simulink model "Att_project_simulink"  (R2022b)
settings: Solver=ode8  StartTime=0.0  StopTime=5000  FixedStep=0.5  RelTol=1e-9  AbsTol=1e-9
values from neighbouring files (symbols this model uses):
  A_R = A_R_BL * ALN_R    [Attitude_proj.m]
  A_T = A_R_BL    [Attitude_proj.m]
  accuracy_earth = deg2rad(10/60)    [Attitude_proj.m]
  accuracy_mag = deg2rad(300/60)    [Attitude_proj.m]
  Cd = 2.3    [Attitude_proj.m]
  I = [Ix 0 0; 0 Iy 0 ; 0 0 Iz]    [Attitude_proj.m]
  Ix = 0.07    [Attitude_proj.m]
  Iy = 0.0504    [Attitude_proj.m]
  Iz = 0.0109    [Attitude_proj.m]
  kd_detum = 2 .* kp_detum    [Attitude_proj.m]
  kd_slew = 2 * kp_slew    [Attitude_proj.m]
  kd_track = kd_detum    [Attitude_proj.m]
  kp_detum = [0.00008 0.0005 0.0005]    [Attitude_proj.m]
  kp_slew = [0.0005 0.0004 0.0004]    [Attitude_proj.m]
  kp_track = kp_detum    [Attitude_proj.m]
  Kx = (Iy-Iz)/Ix    (= 0.564285714286)    [Attitude_proj.m]
  Ky = (Iz-Ix)/Iy    (= -1.17261904762)    [Attitude_proj.m]
  Kz = (Ix-Iy)/Iz    (= 1.79816513761)    [Attitude_proj.m]
  m_para = [0.03;0.04;0.05]    [Attitude_proj.m]
  ortog = (1/3 * deg2rad(1)^2)    [Attitude_proj.m]
  P = Fe/c    (= 4.52980041279e-06)    [Attitude_proj.m]
  q_r = [q1r q2r q3r q4r]    [Attitude_proj.m]
  rho_d_main = 0.1    [Attitude_proj.m]
  rho_d_panel = 0.1    [Attitude_proj.m]
  rho_s_main = 0.5    [Attitude_proj.m]
  rho_s_panel = 0.1    [Attitude_proj.m]
  Rs = 147098074    [Attitude_proj.m]
  w0x = 0.0001    [Attitude_proj.m]
  w0y = orbit.n + 0.005    [Attitude_proj.m]
  w0z = 0.0002    [Attitude_proj.m]
  w_track = [0; orbit.n ; 0]    [Attitude_proj.m]
  zero_w = [ 0; 0; 0]    [Attitude_proj.m]
undefined symbols (not defined in the file or in its folder): body, DiscIntNeverNeededParam, g, h, K, k2, magnitude, orbit, phi0, psi0, theta0, thrus
libraries: vrlib x60, matrix_library x7, simulink x4, sharedutil x4, simulink_extras x2, cstblocks x1, aerolibconvert2 x1, sharedtransform x1
(part 1 of 2)
settings Model: SimulationMode=accelerator  Creator=ASUS  LastModifiedBy=utente
settings SolverCC: ZeroCrossAlgorithm=Adaptive
settings DebuggingCC: AlgebraicLoopMsg=none  MaskedZcDiagnostic=none  IgnoredZcDiagnostic=none  ArithmeticOperatorsInVariantConditions=warning
settings ModelReferenceCC: EnableRefExpFcnMdlSchedulingChecks=on
settings SFSimCC: CustomCodeUndefinedFunction=UseInterfaceOnly
settings RTWCC: DLArmComputeVersion=19.05

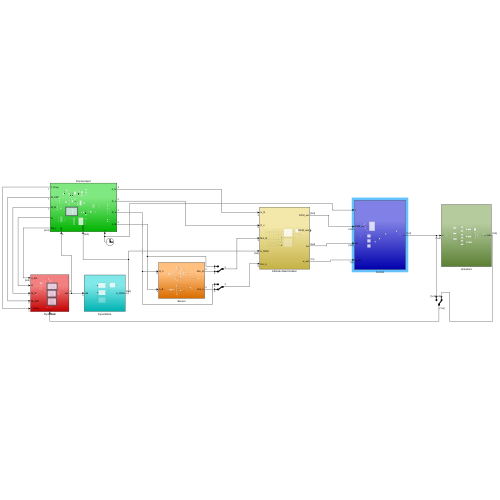
[thumbnail: Simulink's stored preview of the top-level diagram]
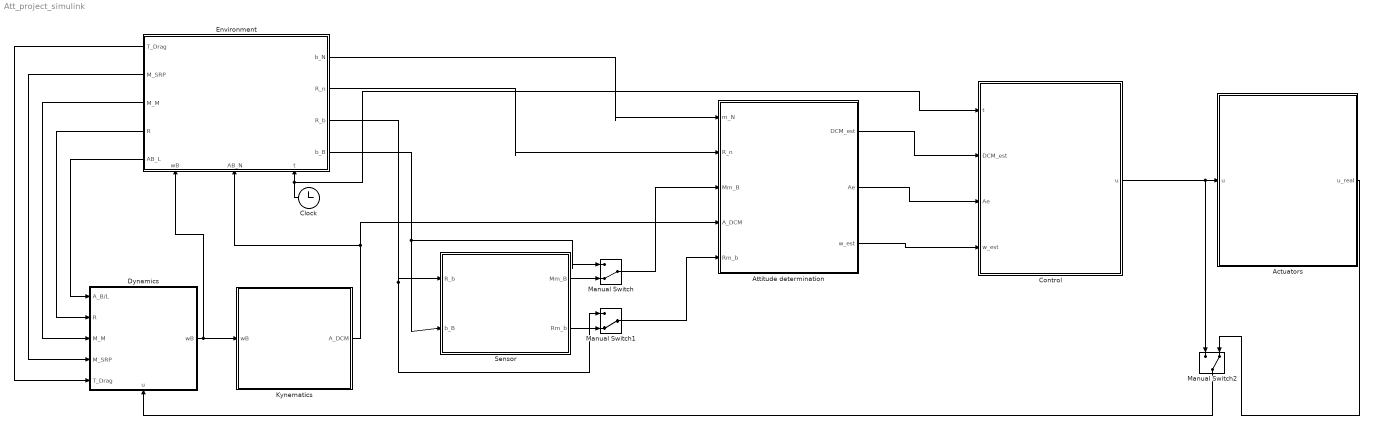
== system Att_project_simulink ==
  Actuators : Subsystem
  Attitude determination : Subsystem
  Clock : Clock
  Control : Subsystem
  Dynamics : Subsystem
      settings: PortSchema="{\"entries\":[{\"content\":{\"sides\":[{\"content\":{\"connectorIds\":[\"In1\",\"In2\",\"In3\",\"In4\",\"In5\"]},\"type\":\"ConnectorPlacement.EquallySpacedRectSide\",\"uuid\":\"e2546f43-0f76-43d8-9016-47189d28d8c0\"},{\"content\":{\"connectorIds\":[\"Out1\"],\"side\":\"RIGHT\"},\"type\":\"ConnectorPlacement.EquallySpacedRectSide\",\"uuid\":\"72ec595a-943a-4b6a-9d51-6626181bb7e6\"},{\"content\":{\"connectorIds\":[],\"side\":\"TOP\"},\"type\":\"ConnectorPlacement.EquallySpacedRectSide\",\"uuid\":\"5bae7898-d8cb-4ebe-a0da-616b512951ce\"},{\"content\":{\"connectorIds\":[\"In6\"],\"side\":\"BOTTOM\"},\"type\":\"ConnectorPlacement.EquallySpacedRectSide\",\"uuid\":\"04644b50-7571-45c4-9210-649b5fcee47a\"}]},\"type\":\"ConnectorPlacement.EquallySpacedConnector\",\"uuid\":\"4d81f698-3eae-4e23-8a75-7ab54dd2047e\"}],\"packageUris\":[\"http://schema.mathworks.com/mf0/Connector/R2020b\"],\"version\":\"1.0\"}"
  Environment : Subsystem
      settings: PortSchema="{\"entries\":[{\"content\":{\"sides\":[{\"content\":{\"connectorIds\":[\"In1\",\"In2\",\"In3\"]},\"type\":\"ConnectorPlacement.EquallySpacedRectSide\",\"uuid\":\"e1717e5b-cb7c-4233-b289-9a3e14a88712\"},{\"content\":{\"connectorIds\":[],\"side\":\"RIGHT\"},\"type\":\"ConnectorPlacement.EquallySpacedRectSide\",\"uuid\":\"74d5df0c-20a5-474c-8972-acb600e0318c\"},{\"content\":{\"connectorIds\":[\"Out5\",\"Out6\",\"Out7\",\"Out8\",\"Out9\"],\"side\":\"TOP\"},\"type\":\"ConnectorPlacement.EquallySpacedRectSide\",\"uuid\":\"8caa1d13-4dab-4013-a60f-fe12337e8062\"},{\"content\":{\"connectorIds\":[\"Out1\",\"Out2\",\"Out3\",\"Out4\"],\"side\":\"BOTTOM\"},\"type\":\"ConnectorPlacement.EquallySpacedRectSide\",\"uuid\":\"a6d0af15-bded-4708-9665-a508da3512a2\"}]},\"type\":\"ConnectorPlacement.EquallySpacedConnector\",\"uuid\":\"6bd2fac6-7248-4b84-8ef8-6b1152c12a45\"}],\"packageUris\":[\"http://schema.mathworks.com/mf0/Connector/R2020b\"],\"version\":\"1.0\"}"
  Kynematics : Subsystem
  Manual Switch : ManualSwitch  CurrentSetting=0
  Manual Switch1 : ManualSwitch  CurrentSetting=0
  Manual Switch2 : ManualSwitch  CurrentSetting=0
  Sensor : Subsystem
  wires:
  Environment/5(AB_L) -> Dynamics/1(A_B/L)
  Environment/6(R) -> Dynamics/2(R)
  Dynamics/1(wB) -> Environment/1(wB), Kynematics/1(wB)
  Environment/7(M_M) -> Dynamics/3(M_M)
  Environment/8(M_SRP) -> Dynamics/4(M_SRP)
  Environment/9(T_Drag) -> Dynamics/5(T_Drag)
  Kynematics/1(A_DCM) -> Environment/2(AB_N), Attitude determination/4(A_DCM)
  Environment/1(b_B) -> Sensor/2(b_B), Manual Switch/1
  Environment/2(R_b) -> Manual Switch1/1, Sensor/1(R_b)
  Sensor/1(Mm_B) -> Manual Switch/2
  Environment/4(b_N) -> Attitude determination/1(m_N)
  Environment/3(R_n) -> Attitude determination/2(R_n)
  Manual Switch/1 -> Attitude determination/3(Mm_B)
  Sensor/2(Rm_b) -> Manual Switch1/2
  Manual Switch1/1 -> Attitude determination/5(Rm_b)
  Clock/1 -> Control/1(t), Environment/3(t)
  Attitude determination/2(Ae) -> Control/3(Ae)
  Control/1(u) -> Manual Switch2/1, Actuators/1(u)
  Attitude determination/1(DCM_est) -> Control/2(DCM_est)
  Attitude determination/3(w_est) -> Control/4(w_est)
  Actuators/1(u_real) -> Manual Switch2/2
  Manual Switch2/1 -> Dynamics/6(u)

== system Att_project_simulink/Actuators ==
  u : Inport
  Demux : Demux  Outputs=3
  If : If
  If Action Subsystem : Subsystem  TreatAsAtomicUnit=on
  If Action Subsystem1 : Subsystem  TreatAsAtomicUnit=on
  If Action Subsystem2 : Subsystem  TreatAsAtomicUnit=on
  If Action Subsystem3 : Subsystem  TreatAsAtomicUnit=on
  If Action Subsystem4 : Subsystem  TreatAsAtomicUnit=on
  If Action Subsystem5 : Subsystem  TreatAsAtomicUnit=on
  If1 : If
  If2 : If
  Merge : Merge
  Merge1 : Merge
  Merge2 : Merge
  Mux : Mux  Inputs=3
  Reshape : Reshape  OutputDimensionality=Customize  OutputDimensions=[1,3]
  Scope : Scope  NumInputPorts=3
  Scope1 : Scope
  To Workspace : ToWorkspace  VariableName=T_c  SaveFormat=Timeseries  SampleTime=-1
  u_real : Outport
  wires:
  u/1 -> Demux/1
  Demux/1 -> If Action Subsystem/1(Mx), If Action Subsystem1/1(-Mx), If/1
  Demux/2 -> If Action Subsystem3/1(-My), If Action Subsystem2/1(My), If1/1
  Demux/3 -> If Action Subsystem5/1(-Mz), If Action Subsystem4/1(Mz), If2/1
  If/1 -> If Action Subsystem/Action
  If/2 -> If Action Subsystem1/Action
  If1/1 -> If Action Subsystem2/Action
  If1/2 -> If Action Subsystem3/Action
  If2/1 -> If Action Subsystem4/Action
  If2/2 -> If Action Subsystem5/Action
  If Action Subsystem4/1(Out1) -> Merge/1  "Z+"
  If Action Subsystem5/1(Out1) -> Merge/2  "Z-"
  If Action Subsystem2/1(Out1) -> Merge1/1  "Y+"
  If Action Subsystem3/1(Out1) -> Merge1/2  "Y-"
  If Action Subsystem/1(Out1) -> Merge2/1  "X+"
  If Action Subsystem1/1(Out1) -> Merge2/2  "X-"
  Mux/1 -> Reshape/1
  Reshape/1 -> Scope1/1, To Workspace/1, u_real/1
  Merge2/1 -> Scope/1, Mux/1
  Merge1/1 -> Scope/2, Mux/2
  Merge/1 -> Scope/3, Mux/3

== system Att_project_simulink/Attitude determination ==
  m_N : Inport
  R_n : Inport  Port=2
  Mm_B : Inport  Port=3
  A_DCM : Inport  Port=4
  Rm_b : Inport  Port=5
  Triad Method : Subsystem
  w_esti : Subsystem
  DCM_est : Outport
  Ae : Outport  Port=2
  w_est : Outport  Port=3
  wires:
  A_DCM/1 -> Triad Method/5(A_DCM)
  Rm_b/1 -> Triad Method/1(Rm_b)
  m_N/1 -> Triad Method/4(m_N)
  Mm_B/1 -> Triad Method/3(Mm_B)
  R_n/1 -> Triad Method/2(R_n)
  Triad Method/1(DCM_est) -> DCM_est/1, w_esti/1(DCM_est)
  Triad Method/2(Ae) -> Ae/1
  w_esti/1(Output) -> w_est/1

== system Att_project_simulink/Control ==
  t : Inport
  DCM_est : Inport  Port=2
  Ae : Inport  Port=3
  w_est : Inport  Port=4
  De-tumbling : Subsystem  Commented=on
  Manual Switch : ManualSwitch  CurrentSetting=0
  Manual Switch1 : ManualSwitch  CurrentSetting=0
  Manual Switch2 : ManualSwitch
  Scope : Scope
  Tracking : Subsystem
  ble : Subsystem  Commented=on
  slew : Subsystem  Commented=on
  w_est1 : InportShadow  Port=4
  u : Outport
  wires:
  Ae/1 -> slew/1(Ae), Tracking/1(Ae), ble/1(Ae)
  [wB] -> ?
  t/1 -> ble/2(t)
  w_est/1 -> ble/3(w_est)
  DCM_est/1 -> ble/4(DCM_est)
  ble/1(u) -> Manual Switch/1
  Manual Switch/1 -> Scope/1, u/1
  w_est1/1 -> De-tumbling/1(In1)
  De-tumbling/1(Out1) -> Manual Switch1/1
  Tracking/1(u) -> Manual Switch2/1
  Manual Switch1/1 -> Manual Switch/2
  slew/1(u) -> Manual Switch2/2
  Manual Switch2/1 -> Manual Switch1/2

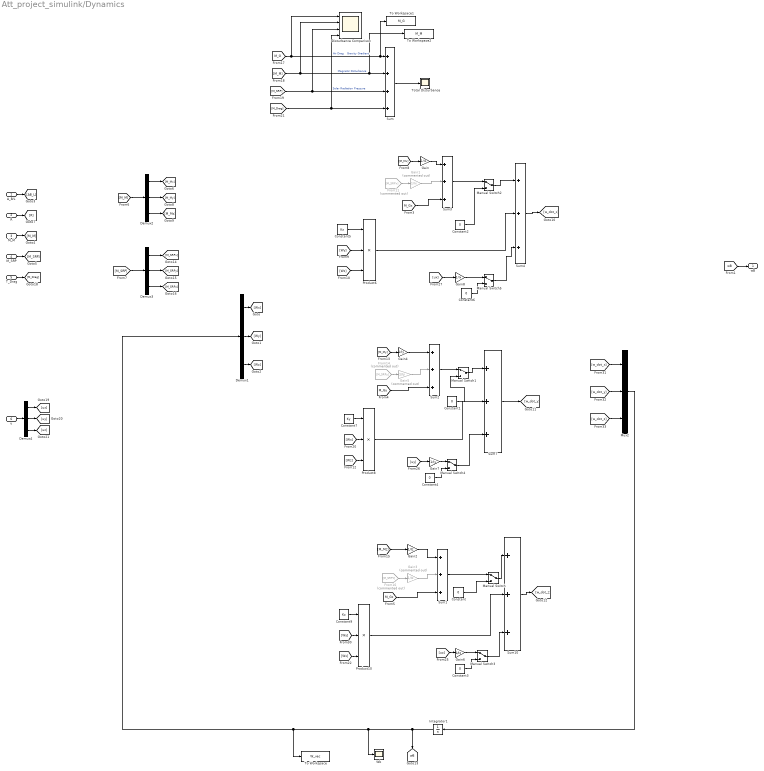
== system Att_project_simulink/Dynamics ==
  A_B/L : Inport
  R : Inport  Port=2
  M_M : Inport  Port=3
  M_SRP : Inport  Port=4
  T_Drag : Inport  Port=5
  u : Inport  Port=6
  Constant{,1..4,6} (6 alike) : Constant  Value=0
  Constant5 : Constant  Value=Kx
  Constant7 : Constant  Value=Ky
  Constant9 : Constant  Value=Kz
  Demux{1..4} (4 alike) : Demux  Outputs=3
  Disturbance Comparison : Scope  NumInputPorts=4
  From11 : From  Commented=on  GotoTag=M_SRPx
  From14 : From  Commented=on  GotoTag=M_SRPy
  From16 : From  Commented=on  GotoTag=M_SRPz
  Gain : Gain  Gain=1/Ix
  Gain1 : Gain  Commented=on  Gain=1/Ix
  Gain2 : Gain  Gain=1/Iz
  Gain3 : Gain  Commented=on  Gain=1/Iz
  Gain4 : Gain  Gain=1/Iy
  Gain5 : Gain  Commented=on  Gain=1/Iy
  Gain6 : Gain  Gain=1/Iz
  Gain7 : Gain  Gain=1/Iy
  Gain8 : Gain  Gain=1/Ix
  Integrator1 : Integrator  InitialCondition=[w0x; w0y; w0z]'
  Manual Switch{,1..5} (6 alike) : ManualSwitch
  Mux2 : Mux  Inputs=3
  Product10 : Product  Inputs=3
  Product6 : Product  Inputs=3
  Product8 : Product  Inputs=3
  Sum : Sum  Inputs=++++
  Sum{1..4,7,10} (6 alike) : Sum  Inputs=+++
  To Workspace : ToWorkspace  VariableName=W_vec  SaveFormat=Timeseries  SampleTime=-1
  To Workspace1 : ToWorkspace  VariableName=M_G  SaveFormat=Timeseries  SampleTime=-1
  To Workspace2 : ToWorkspace  VariableName=M_M  SaveFormat=Timeseries  SampleTime=-1
  Total Disturbance : Scope
  Wb : Scope
  wB : Outport
  tag scope: wB=global
  wires:
  Demux1/3 -> [Wz]
  Demux1/2 -> [Wy]
  Demux1/1 -> [Wx]
  A_B/L/1 -> [AB_L]
  [Wy] -> Product6/2
  [Wz] -> Product6/3
  Product6/1 -> Sum4/2
  Sum4/1 -> [w_dot_x]
  Product8/1 -> Sum7/2
  [Wx] -> Product8/2
  Sum7/1 -> [w_dot_y]
  [Wz] -> Product8/3
  Product10/1 -> Sum10/2
  [Wy] -> Product10/2
  Constant9/1 -> Product10/1
  Sum10/1 -> [w_dot_z]
  [Wx] -> Product10/3
  [w_dot_z] -> Mux2/3
  [w_dot_y] -> Mux2/2
  [w_dot_x] -> Mux2/1
  Integrator1/1 -> Wb/1, To Workspace/1, Demux1/1, [wB]
  Constant5/1 -> Product6/1
  Constant7/1 -> Product8/1
  [wB] -> wB/1
  R/1 -> [R]
  M_M/1 -> [M_M]
  M_SRP/1 -> [M_SRP]
  Demux2/1 -> [M_Mx]
  Demux2/2 -> [M_My]
  Demux2/3 -> [M_Mz]
  [M_M] -> Demux2/1
  Demux3/2 -> [M_SRPy]
  Demux3/1 -> [M_SRPx]
  [M_SRP] -> Demux3/1
  Demux3/3 -> [M_SRPz]
  [M_Mx] -> Gain/1
  From11/1 -> Gain1/1
  [M_My] -> Gain4/1
  From14/1 -> Gain5/1
  From16/1 -> Gain3/1
  [M_Mz] -> Gain2/1
  [M_SRP] -> Sum/3, Disturbance Comparison/3  "Solar Radiation Pressure"
  [M_M] -> To Workspace2/1, Sum/2, Disturbance Comparison/2  "Magnetic Disturbance"
  [M_G] -> Disturbance Comparison/1, To Workspace1/1, Sum/1  "Gravity Gradient"
  Sum/1 -> Total Disturbance/1
  T_Drag/1 -> [M_Drag]
  [M_Drag] -> Sum/4, Disturbance Comparison/4  "Air Drag"
  Gain2/1 -> Sum1/1
  Gain3/1 -> Sum1/2
  [M_Gz] -> Sum1/3
  Sum1/1 -> Manual Switch/1
  Constant/1 -> Manual Switch/2
  Gain4/1 -> Sum2/1
  Gain5/1 -> Sum2/2
  [M_Gy] -> Sum2/3
  Sum2/1 -> Manual Switch1/1
  Manual Switch1/1 -> Sum7/1
  Constant1/1 -> Manual Switch1/2
  Manual Switch/1 -> Sum10/1
  Gain1/1 -> Sum3/2
  Gain/1 -> Sum3/1
  [M_Gx] -> Sum3/3
  Sum3/1 -> Manual Switch2/1
  Manual Switch2/1 -> Sum4/1
  Constant2/1 -> Manual Switch2/2
  Manual Switch3/1 -> Sum10/3
  Constant3/1 -> Manual Switch3/2
  u/1 -> Demux4/1
  Demux4/1 -> [ux]
  Demux4/2 -> [uy]
  Demux4/3 -> [uz]
  [uz] -> Gain6/1
  Constant4/1 -> Manual Switch4/2
  Manual Switch4/1 -> Sum7/3
  [uy] -> Gain7/1
  Constant6/1 -> Manual Switch5/2
  Manual Switch5/1 -> Sum4/3
  [ux] -> Gain8/1
  Gain6/1 -> Manual Switch3/1
  Gain7/1 -> Manual Switch4/1
  Gain8/1 -> Manual Switch5/1
  Mux2/1 -> Integrator1/1

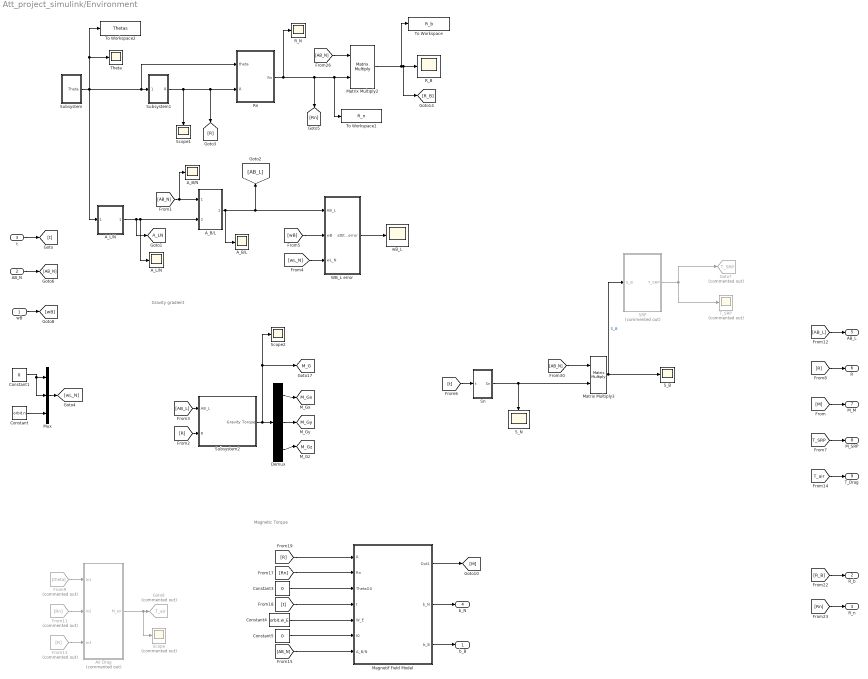
== system Att_project_simulink/Environment ==
  note: Gravity gradient
  note: Magnetic Torque
  wB : Inport
  AB_N : Inport  Port=2
  t : Inport  Port=3
  A_B/L : Scope
  "A_B/L " : Subsystem
  A_B/N : Scope
  A_L/N : Scope
  "A_L/N " : Subsystem
  "Air Drag " : Subsystem  Commented=on
  Constant : Constant  Value=orbit.n
  Constant1 : Constant  Value=0
  Constant3 : Constant  Value=0
  Constant4 : Constant  Value=orbit.w_E
  Constant5 : Constant  Value=0
  Demux : Demux  Outputs=3
  From11 : From  Commented=on  GotoTag=Rn
  From13 : From  Commented=on  GotoTag=R
  From9 : From  Commented=on  GotoTag=theta
  Goto7 : Goto  Commented=on  GotoTag=T_SRP  TagVisibility=global
  Goto9 : Goto  Commented=on  GotoTag=T_air  TagVisibility=global
  Magnetif Field Model : Subsystem
  Matrix Multiply2 : Product  Multiplication=Matrix(*)
  Matrix Multiply3 : Product  Multiplication=Matrix(*)
  Mux : Mux  Inputs=3
  R_B : Scope
  R_N : Scope
  Rn : Subsystem
  SRP : Subsystem  Commented=on
  S_B : Scope
  S_N : Scope
  Scope : Scope  Commented=on
  Scope1 : Scope
  Scope2 : Scope
  Sn : Subsystem
  Subsystem : Subsystem
  Subsystem1 : Subsystem
  Subsystem2 : Subsystem
  T_SRP : Scope  Commented=on
  Theta : Scope
  To Workspace : ToWorkspace  VariableName=R_b  SaveFormat=Timeseries  SampleTime=-1
  To Workspace1 : ToWorkspace  VariableName=R_n  SaveFormat=Timeseries  SampleTime=-1
  To Workspace2 : ToWorkspace  VariableName=Thetas  SaveFormat=Timeseries  SampleTime=-1
  WB_L error : Subsystem
  wB_L : Scope
  b_B : Outport
  R_b : Outport  Port=2
  R_n : Outport  Port=3
  b_N : Outport  Port=4
  AB_L : Outport  Port=5
  R : Outport  Port=6
  M_M : Outport  Port=7
  M_SRP : Outport  Port=8
  T_Drag : Outport  Port=9
  tag scope: A_LN=global, M_G=global, M_Gx=global, M_Gy=global, M_Gz=global
  wires:
  t/1 -> [t]
  Constant/1 -> Mux/3
  Mux/1 -> [wL_N]
  AB_N/1 -> [AB_N]
  [AB_L] -> AB_L/1
  Matrix Multiply2/1 -> To Workspace/1, [R_B], R_B/1
  Subsystem/1(Theta) -> Rn/1(theta), Subsystem1/1(Theta), To Workspace2/1, Theta/1, "A_L/N "/1(theta)
  [AB_N] -> A_B/N/1, "A_B/L "/1(AB_N)
  "A_L/N "/1(AL_N) -> [A_LN], "A_B/L "/2(AL_N), A_L/N/1
  WB_L error/1(attitude error) -> wB_L/1
  "A_B/L "/1(AB_L) -> A_B/L/1, WB_L error/1(AB_L), [AB_L]
  [wL_N] -> WB_L error/3(wL_N)
  Subsystem1/1(R) -> Scope1/1, Rn/2(R), [R]
  [R] -> R/1
  Rn/1(Rn) -> R_N/1, To Workspace1/1, Matrix Multiply2/2, [Rn]
  [AB_N] -> Matrix Multiply2/1
  Constant1/1 -> Mux/2, Mux/1
  wB/1 -> [wB]
  [wB] -> WB_L error/2(wB)
  [T_SRP] -> M_SRP/1
  [M] -> M_M/1
  From9/1 -> "Air Drag "/1(In1)
  From11/1 -> "Air Drag "/2(In2)
  From13/1 -> "Air Drag "/3(In3)
  "Air Drag "/1(M_air) -> Scope/1, Goto9/1
  [T_air] -> T_Drag/1
  [Rn] -> Magnetif Field Model/2(Rn)
  Constant3/1 -> Magnetif Field Model/3(ThetaG0)
  [t] -> Magnetif Field Model/4(t)
  Constant4/1 -> Magnetif Field Model/5(W_E)
  Constant5/1 -> Magnetif Field Model/6(t0)
  [AB_N] -> Magnetif Field Model/7(A_B/N)
  [R] -> Magnetif Field Model/1(R)
  Magnetif Field Model/1(Out1) -> [M]
  [t] -> Sn/1(t)
  Sn/1(Sn) -> Matrix Multiply3/2, S_N/1
  Matrix Multiply3/1 -> SRP/1(S_B), S_B/1  "S_B"
  SRP/1(T_SRP) -> T_SRP/1, Goto7/1
  [AB_N] -> Matrix Multiply3/1
  Magnetif Field Model/2(b_N) -> b_N/1
  Magnetif Field Model/3(b_B) -> b_B/1
  [R_B] -> R_b/1
  [Rn] -> R_n/1
  [R] -> Subsystem2/2(R)
  Subsystem2/1(Gravity Torque) -> Scope2/1, [M_G], Demux/1
  Demux/2 -> [M_Gy]
  Demux/3 -> [M_Gz]
  [AB_L] -> Subsystem2/1(AB_L)
  Demux/1 -> [M_Gx]

== system Att_project_simulink/Kynematics ==
  wB : Inport
  DCM : Subsystem
  Euler Angles : Subsystem  Commented=on
  From Quat to DCM : Subsystem
  Quaternions : Subsystem
  A_DCM : Outport
  wires:
  Quaternions/1(q(t)) -> From Quat to DCM/1(q(t))
  From Quat to DCM/1(A_DCM) -> A_DCM/1
  wB/1 -> Euler Angles/1(wB), DCM/1(wB), Quaternions/1(wB)
  DCM/1(dcm) -> From Quat to DCM/2(dcm)

== system Att_project_simulink/Sensor ==
  R_b : Inport
  b_B : Inport  Port=2
  Demux : Demux  Outputs=3
  Demux1 : Demux  Outputs=3
  Mux : Mux  Inputs=3
  Mux1 : Mux  Inputs=3
  Normalize Vector : vrlib/Utilities/Normalize Vector  maxzero=0
  Normalize Vector1 : vrlib/Utilities/Normalize Vector  maxzero=0
  Random Number1 : RandomNumber  Variance=(1/3*accuracy_mag).^2  Seed=1  SampleTime=1
  Random Number10 : RandomNumber  Variance=ortog  Seed=2  SampleTime=2
  Random Number11 : RandomNumber  Variance=ortog  Seed=3  SampleTime=2
  Random Number2 : RandomNumber  Variance=(1/3*accuracy_mag).^2  Seed=2  SampleTime=1
  Random Number3 : RandomNumber  Variance=(1/3*accuracy_mag).^2  Seed=3  SampleTime=1
  Random Number4 : RandomNumber  Variance=(1/3*accuracy_earth).^2  Seed=4  SampleTime=2
  Random Number7 : RandomNumber  Variance=(1/3*accuracy_earth).^2  Seed=5  SampleTime=2
  Random Number8 : RandomNumber  Variance=(1/3*accuracy_earth).^2  Seed=6  SampleTime=2
  Random Number9 : RandomNumber  Variance=ortog  Seed=1  SampleTime=2
  Reshape : Reshape  OutputDimensionality=Customize  OutputDimensions=[3,1]
  Reshape1 : Reshape  OutputDimensionality=Customize  OutputDimensions=[3,1]
  Scope3 : Scope  NumInputPorts=2
  Scope4 : Scope  NumInputPorts=2
  Sum1 : Sum  Inputs=+++
  Sum2 : Sum  Inputs=+++
  Sum3 : Sum  Inputs=+++
  Sum4 : Sum  Inputs=++|
  Sum5 : Sum  Inputs=|++
  Sum6 : Sum  Inputs=|++
  Mm_B : Outport
  Rm_b : Outport  Port=2
  wires:
  Random Number1/1 -> Sum1/1
  Demux/3 -> Sum3/1
  Random Number3/1 -> Sum3/2
  Sum1/1 -> Mux/1
  Sum2/1 -> Mux/2
  Sum3/1 -> Mux/3
  Demux1/2 -> Sum5/1
  Random Number7/1 -> Sum5/2
  Demux1/3 -> Sum6/1
  Random Number8/1 -> Sum6/2
  Random Number4/1 -> Sum4/1
  Sum4/1 -> Mux1/1
  Sum6/1 -> Mux1/3
  Demux1/1 -> Sum4/2
  Sum5/1 -> Mux1/2
  Mux1/1 -> Scope3/2, Rm_b/1
  R_b/1 -> Normalize Vector/1
  Normalize Vector/1 -> Reshape1/1
  Normalize Vector1/1 -> Reshape/1
  Mux/1 -> Mm_B/1, Scope4/1
  b_B/1 -> Normalize Vector1/1
  Demux/1 -> Sum1/3
  Random Number9/1 -> Sum1/2
  Random Number2/1 -> Sum2/1
  Random Number10/1 -> Sum2/2
  Demux/2 -> Sum2/3
  Random Number11/1 -> Sum3/3
  Reshape/1 -> Scope4/2, Demux/1
  Reshape1/1 -> Scope3/1, Demux1/1

== system Att_project_simulink/Actuators/If Action Subsystem ==
  Mx : Inport
  Action Port : ActionPort  ActionPortLabel=if(u1 > 0)
  Abs : Abs  SaturateOnIntegerOverflow=off
  Constant : Constant  Value=thrus.ACT_x1(3)
  Divide : Product  Inputs=*/
  Product : Product
  Saturation : Saturate  UpperLimit=thrus.up_sat  LowerLimit=thrus.low_sat
  Out1 : Outport
  wires:
  Mx/1 -> Divide/1
  Constant/1 -> Abs/1
  Divide/1 -> Saturation/1
  Saturation/1 -> Product/2
  Product/1 -> Out1/1
  Abs/1 -> Product/1, Divide/2

== system Att_project_simulink/Actuators/If Action Subsystem1 ==
  -Mx : Inport
  Action Port : ActionPort  ActionPortLabel=else
  Abs : Abs  SaturateOnIntegerOverflow=off
  Constant : Constant  Value=thrus.ACT_x2(3)
  Divide : Product  Inputs=*/
  Gain : Gain  Gain=-1
  Gain1 : Gain  Gain=-1
  Product : Product
  Saturation : Saturate  UpperLimit=thrus.up_sat  LowerLimit=thrus.low_sat
  Scope : Scope  NumInputPorts=2
  Out1 : Outport
  wires:
  Saturation/1 -> Scope/2, Product/2
  Product/1 -> Gain1/1
  Constant/1 -> Abs/1
  Divide/1 -> Scope/1, Saturation/1
  -Mx/1 -> Gain/1
  Abs/1 -> Product/1, Divide/2
  Gain/1 -> Divide/1
  Gain1/1 -> Out1/1

== system Att_project_simulink/Actuators/If Action Subsystem2 ==
  My : Inport
  Action Port : ActionPort  ActionPortLabel=if(u1 > 0)
  Abs : Abs  SaturateOnIntegerOverflow=off
  Constant : Constant  Value=thrus.ACT_y1(3)
  Divide : Product  Inputs=*/
  Product : Product
  Saturation : Saturate  UpperLimit=thrus.up_sat  LowerLimit=thrus.low_sat
  Out1 : Outport
  wires:
  Saturation/1 -> Product/2
  Product/1 -> Out1/1
  Constant/1 -> Abs/1
  Divide/1 -> Saturation/1
  My/1 -> Divide/1
  Abs/1 -> Product/1, Divide/2

== system Att_project_simulink/Actuators/If Action Subsystem3 ==
  -My : Inport
  Action Port : ActionPort  ActionPortLabel=else
  Abs : Abs  SaturateOnIntegerOverflow=off
  Constant : Constant  Value=thrus.ACT_y2(3)
  Divide : Product  Inputs=*/
  Gain : Gain  Gain=-1
  Gain1 : Gain  Gain=-1
  Product : Product
  Saturation : Saturate  UpperLimit=thrus.up_sat  LowerLimit=thrus.low_sat
  Out1 : Outport
  wires:
  Saturation/1 -> Product/2
  Product/1 -> Gain1/1
  Constant/1 -> Abs/1
  Divide/1 -> Saturation/1
  -My/1 -> Gain/1
  Abs/1 -> Product/1, Divide/2
  Gain/1 -> Divide/1
  Gain1/1 -> Out1/1

== system Att_project_simulink/Actuators/If Action Subsystem4 ==
  Mz : Inport
  Action Port : ActionPort  ActionPortLabel=if(u1 > 0)
  Abs : Abs  SaturateOnIntegerOverflow=off
  Constant : Constant  Value=thrus.ACT_z1(2)
  Divide : Product  Inputs=*/
  Product : Product
  Saturation : Saturate  UpperLimit=thrus.up_sat  LowerLimit=thrus.low_sat
  Out1 : Outport
  wires:
  Saturation/1 -> Product/2
  Product/1 -> Out1/1
  Constant/1 -> Abs/1
  Divide/1 -> Saturation/1
  Mz/1 -> Divide/1
  Abs/1 -> Product/1, Divide/2

== system Att_project_simulink/Actuators/If Action Subsystem5 ==
  -Mz : Inport
  Action Port : ActionPort  ActionPortLabel=else
  Abs : Abs  SaturateOnIntegerOverflow=off
  Constant : Constant  Value=thrus.ACT_z2(2)
  Divide : Product  Inputs=*/
  Gain : Gain  Gain=-1
  Gain1 : Gain  Gain=-1
  Product : Product
  Saturation : Saturate  UpperLimit=thrus.up_sat  LowerLimit=thrus.low_sat
  Out1 : Outport
  wires:
  Saturation/1 -> Product/2
  Product/1 -> Gain1/1
  Constant/1 -> Abs/1
  Divide/1 -> Saturation/1
  -Mz/1 -> Gain/1
  Abs/1 -> Product/1, Divide/2
  Gain/1 -> Divide/1
  Gain1/1 -> Out1/1

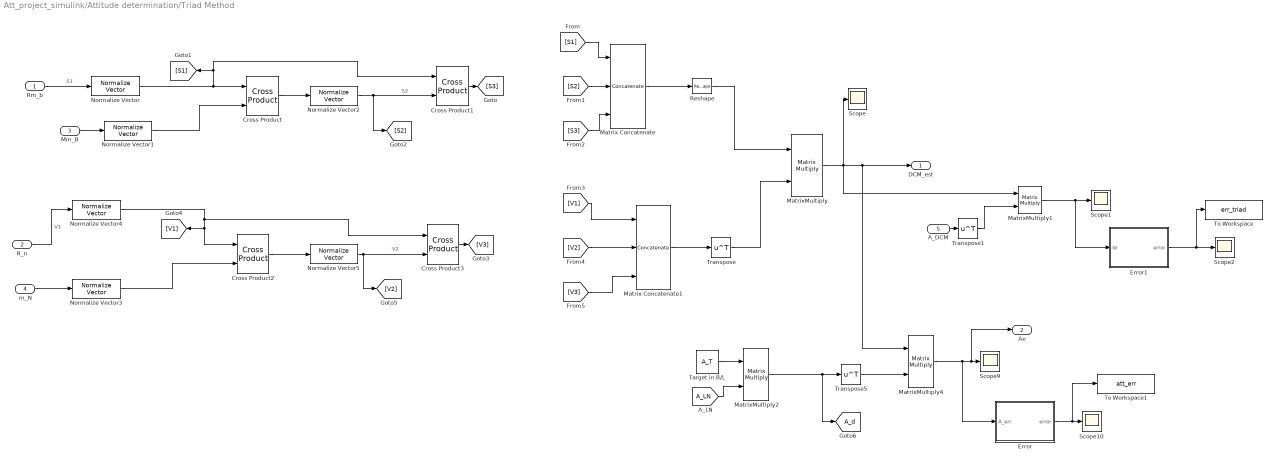
== system Att_project_simulink/Attitude determination/Triad Method ==
  Rm_b : Inport
  R_n : Inport  Port=2
  Mm_B : Inport  Port=3
  m_N : Inport  Port=4
  A_DCM : Inport  Port=5
  Cross Product{,1..3} (4 alike) : matrix_library/Cross Product
  Error : Subsystem
  Error1 : Subsystem
  Matrix Concatenate : Concatenate  NumInputs=3  Mode=Multidimensional array  ConcatenateDimension=2
  Matrix Concatenate1 : Concatenate  NumInputs=3  Mode=Multidimensional array  ConcatenateDimension=2
  MatrixMultiply{,1..2,4} (4 alike) : Product  Multiplication=Matrix(*)
  Normalize Vector{,1..5} (6 alike) : vrlib/Utilities/Normalize Vector  maxzero=0
  Reshape : Reshape  OutputDimensionality=Customize  OutputDimensions=[3,3]
  Scope{,1..2,9..10} (5 alike) : Scope
  Target in B/L : Constant  Value=A_T  VectorParams1D=off
  To Workspace : ToWorkspace  VariableName=err_triad  SaveFormat=Structure  SampleTime=-1
  To Workspace1 : ToWorkspace  VariableName=att_err  SaveFormat=Timeseries  SampleTime=-1
  Transpose : Math  Operator=transpose
  Transpose1 : Math  Operator=transpose
  Transpose5 : Math  Operator=transpose
  DCM_est : Outport
  Ae : Outport  Port=2
  tag scope: A_d=global
  wires:
  Rm_b/1 -> Normalize Vector/1  "S1"
  Cross Product/1 -> Normalize Vector2/1
  Normalize Vector2/1 -> [S2], Cross Product1/2  "S2"
  Cross Product1/1 -> [S3]
  m_N/1 -> Normalize Vector3/1
  Cross Product3/1 -> [V3]
  Cross Product2/1 -> Normalize Vector5/1
  R_n/1 -> Normalize Vector4/1  "V1"
  Normalize Vector5/1 -> [V2], Cross Product3/2  "V2"
  [S1] -> Matrix Concatenate/1
  [S2] -> Matrix Concatenate/2
  [S3] -> Matrix Concatenate/3
  [V1] -> Matrix Concatenate1/1
  [V2] -> Matrix Concatenate1/2
  [V3] -> Matrix Concatenate1/3
  Matrix Concatenate1/1 -> Transpose/1
  Transpose/1 -> MatrixMultiply/2
  MatrixMultiply/1 -> DCM_est/1, MatrixMultiply4/1, MatrixMultiply1/1, Scope/1
  A_DCM/1 -> Transpose1/1
  Transpose1/1 -> MatrixMultiply1/2
  MatrixMultiply1/1 -> Error1/1(Id), Scope1/1
  Normalize Vector/1 -> [S1], Cross Product1/1, Cross Product/1
  Mm_B/1 -> Normalize Vector1/1
  Normalize Vector1/1 -> Cross Product/2
  Normalize Vector4/1 -> Cross Product2/1, [V1], Cross Product3/1
  Normalize Vector3/1 -> Cross Product2/2
  Transpose5/1 -> MatrixMultiply4/2
  MatrixMultiply4/1 -> Error/1(A_err), Ae/1, Scope9/1
  Error/1(error) -> To Workspace1/1, Scope10/1
  Error1/1(error) -> To Workspace/1, Scope2/1
  Target in B/L/1 -> MatrixMultiply2/1
  [A_LN] -> MatrixMultiply2/2
  Matrix Concatenate/1 -> Reshape/1
  Reshape/1 -> MatrixMultiply/1
  MatrixMultiply2/1 -> [A_d], Transpose5/1

== system Att_project_simulink/Attitude determination/w_esti ==
  DCM_est : Inport
  Constant : Constant  Value=0.2
  Discrete Derivative : simulink/Quick Insert/Discrete/Discrete Derivative  gainval=1.0  ICPrevScaledInput=0.0  OutMin=[]  OutMax=[]  OutDataType=fixdt(1, 16)  OutScaling=2^-10  DoSatur=off
  Discrete Varying Lowpass : cstblocks/Linear Parameter Varying/Discrete Varying Lowpass  N=5  w0=0  Ts=1
  Gain : Gain  Gain=-1
  MATLAB Function : MATLAB Function  TreatAsAtomicUnit=on
  Manual Switch1 : ManualSwitch
  MatrixMultiply : Product  Multiplication=Matrix(*)
  Scope : Scope  NumInputPorts=2
  Scope1 : Scope
  Scope2 : Scope
  Sum : Sum  Inputs=|+-
  Transpose : Math  Operator=transpose
  Output : Outport
  wires:
  DCM_est/1 -> Discrete Derivative/1, Transpose/1
  [wB] -> Scope2/1, Scope/2, Sum/2
  Sum/1 -> Scope1/1
  Gain/1 -> MATLAB Function/1(w)
  MatrixMultiply/1 -> Gain/1  "-w"
  Discrete Derivative/1 -> MatrixMultiply/1
  Transpose/1 -> MatrixMultiply/2
  MATLAB Function/1(w_est) -> Manual Switch1/2, Discrete Varying Lowpass/1
  Discrete Varying Lowpass/1 -> Manual Switch1/1
  Manual Switch1/1 -> Sum/1, Output/1, Scope/1
  Constant/1 -> Discrete Varying Lowpass/2

== system Att_project_simulink/Control/De-tumbling ==
  In1 : Inport
  Constant : Constant  Value=zero_w
  Discrete Derivative : simulink/Discrete/Discrete Derivative  gainval=1.0  ICPrevScaledInput=0.0  OutMin=[]  OutMax=[]  OutDataType=fixdt(1, 16)  OutScaling=2^-10  DoSatur=off
  Discrete-Time Integrator : DiscreteIntegrator  SampleTime=-1  ICPrevOutput=DiscIntNeverNeededParam  ICPrevScaledInput=DiscIntNeverNeededParam
  Gain : Gain  Gain=-kp_detum
  Gain1 : Gain  Gain=-kd_detum
  Gain2 : Gain  Gain=-kp_detum
  Reshape : Reshape  OutputDimensionality=Customize  OutputDimensions=[1,3]
  Reshape1 : Reshape  OutputDimensionality=Customize  OutputDimensions=[1,3]
  Sum : Sum  Inputs=+++
  Sum1 : Sum  Inputs=|++
  Out1 : Outport
  wires:
  In1/1 -> Reshape/1
  Discrete Derivative/1 -> Gain1/1
  Sum/1 -> Reshape1/1
  Reshape/1 -> Discrete-Time Integrator/1, Gain/1, Discrete Derivative/1
  Reshape1/1 -> Out1/1
  Gain/1 -> Sum1/1
  Constant/1 -> Sum1/2
  Sum1/1 -> Sum/2
  Gain1/1 -> Sum/3
  Discrete-Time Integrator/1 -> Gain2/1
  Gain2/1 -> Sum/1

== system Att_project_simulink/Control/Tracking ==
  Ae : Inport
  Constant : Constant  Value=w_track
  Discrete Derivative : simulink/Discrete/Discrete Derivative  gainval=1.0  ICPrevScaledInput=0.0  OutMin=[]  OutMax=[]  OutDataType=fixdt(1, 16)  OutScaling=2^-10  DoSatur=off
  Gain : Gain  Gain=-kp_track
  Gain1 : Gain  Gain=-kd_track
  Mux : Mux  Inputs=3
  Scope : Scope
  Selector : Selector  NumberOfDimensions=2  InputPortWidth=3  IndexOptions=Index vector (dialog),Index vector (dialog)  Indices=2,3  OutputSizes=1,1
  Selector1 : Selector  NumberOfDimensions=2  InputPortWidth=3  IndexOptions=Index vector (dialog),Index vector (dialog)  Indices=3,1  OutputSizes=1,1
  Selector2 : Selector  NumberOfDimensions=2  InputPortWidth=3  IndexOptions=Index vector (dialog),Index vector (dialog)  Indices=1,2  OutputSizes=1,1
  Sum : Sum  Inputs=|++
  Sum1 : Sum  Inputs=|+-
  u : Outport
  wires:
  Selector/1 -> Mux/1
  Selector2/1 -> Mux/3
  Gain1/1 -> Sum/1
  Gain/1 -> Sum/2
  Selector1/1 -> Mux/2
  Discrete Derivative/1 -> Sum1/1, Scope/1
  Constant/1 -> Sum1/2
  Sum1/1 -> Gain1/1
  Mux/1 -> Gain/1, Discrete Derivative/1
  Sum/1 -> u/1
  Ae/1 -> Selector/1, Selector2/1, Selector1/1

== system Att_project_simulink/Control/ble ==
  Ae : Inport
  t : Inport  Port=2
  w_est : Inport  Port=3
  DCM_est : Inport  Port=4
  Constant1 : Constant  Value=I
  Demux : Demux  Outputs=9
  Extract Diagonal : matrix_library/Extract Diagonal
      settings: LibrarySourceBlock=|
      | simulink/Matrix
      | Operations/Extract Diagonal
  Gain1 : Gain  Gain=k2
  Gain2 : Gain  Gain=-kd_track
  Gain3 : Gain  Gain=-kp_track
  Gain4 : Gain  Gain=0.5
  MatrixMultiply : Product  Multiplication=Matrix(*)
  MatrixMultiply1 : Product  Multiplication=Matrix(*)
  Reshape : Reshape  OutputDimensionality=Customize  OutputDimensions=[9,1]
  Reshape1 : Reshape  OutputDimensionality=Customize  OutputDimensions=[1,3]
  Reshape2 : Reshape  OutputDimensionality=Customize  OutputDimensions=[1,3]
  Scope : Scope  NumInputPorts=2
  Scope2 : Scope
  Sum : Sum  Inputs=|+-
  Sum of Elements : Sum  Inputs=+
  Sum1 : Sum  Inputs=|++
  Sum2 : Sum  Inputs=|++
  Sum3 : Sum  Inputs=|+-
  Transpose : Math  Operator=transpose
  Transpose1 : Math  Operator=transpose
  Vector Concatenate : Concatenate  NumInputs=3
  u : Outport
  wires:
  Ae/1 -> Sum/2, Transpose/1
  Transpose/1 -> Sum/1
  Sum/1 -> Reshape/1
  Reshape/1 -> Demux/1
  Demux/7 -> Vector Concatenate/2
  Demux/6 -> Vector Concatenate/1
  Demux/2 -> Vector Concatenate/3
  Vector Concatenate/1 -> Reshape1/1
  Gain2/1 -> Sum1/1
  Gain3/1 -> Sum1/2
  Reshape1/1 -> Scope/1, Gain2/1
  w_est/1 -> Reshape2/1, Transpose1/1, MatrixMultiply1/2
  Reshape2/1 -> Gain3/1
  Sum1/1 -> u/1, Scope/2
  Transpose1/1 -> MatrixMultiply/1
  Constant1/1 -> MatrixMultiply/2
  MatrixMultiply1/1 -> Gain4/1
  MatrixMultiply/1 -> MatrixMultiply1/1
  Extract Diagonal/1 -> Sum of Elements/1
  Sum of Elements/1 -> Gain1/1
  [A_d] -> Sum3/1
  DCM_est/1 -> Sum3/2
  Sum3/1 -> Extract Diagonal/1
  Gain1/1 -> Sum2/2
  Sum2/1 -> Scope2/1
  Gain4/1 -> Sum2/1

== system Att_project_simulink/Control/slew ==
  Ae : Inport
  Discrete Derivative : simulink/Discrete/Discrete Derivative  gainval=1.0  ICPrevScaledInput=0.0  OutMin=[]  OutMax=[]  OutDataType=fixdt(1, 16)  OutScaling=2^-10  DoSatur=off
  Gain : Gain  Gain=-kp_slew
  Gain1 : Gain  Gain=-kd_slew
  Mux : Mux  Inputs=3
  Scope : Scope
  Selector : Selector  NumberOfDimensions=2  InputPortWidth=3  IndexOptions=Index vector (dialog),Index vector (dialog)  Indices=2,3  OutputSizes=1,1
  Selector1 : Selector  NumberOfDimensions=2  InputPortWidth=3  IndexOptions=Index vector (dialog),Index vector (dialog)  Indices=3,1  OutputSizes=1,1
  Selector2 : Selector  NumberOfDimensions=2  InputPortWidth=3  IndexOptions=Index vector (dialog),Index vector (dialog)  Indices=1,2  OutputSizes=1,1
  Sum : Sum  Inputs=|++
  u : Outport
  wires:
  Sum/1 -> u/1
  Mux/1 -> Discrete Derivative/1, Gain/1
  Discrete Derivative/1 -> Gain1/1, Scope/1
  Selector1/1 -> Mux/2
  Gain/1 -> Sum/2
  Gain1/1 -> Sum/1
  Selector2/1 -> Mux/3
  Selector/1 -> Mux/1
  Ae/1 -> Selector/1, Selector1/1, Selector2/1

== system Att_project_simulink/Environment/A_B//L  ==
  AB_N : Inport
  AL_N : Inport  Port=2
  Matrix Multiply : Product  Multiplication=Matrix(*)
  Transpose : Math  Operator=transpose
  AB_L : Outport
  wires:
  [AL_N] -> Transpose/1
  Matrix Multiply/1 -> [AB_L]
  [AB_N] -> Matrix Multiply/1
  Transpose/1 -> Matrix Multiply/2
  [AB_L] -> AB_L/1
  AL_N/1 -> [AL_N]
  AB_N/1 -> [AB_N]

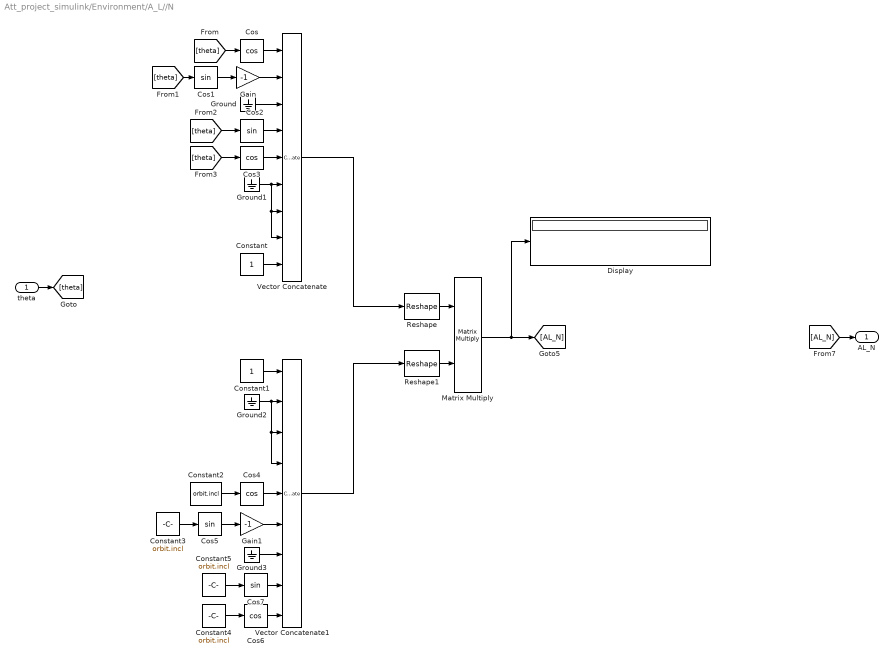
== system Att_project_simulink/Environment/A_L//N  ==
  theta : Inport
  Constant : Constant
  Constant1 : Constant
  Constant{2..5} (4 alike) : Constant  Value=orbit.incl
  Cos{,3..4,6} (4 alike) : Trigonometry  Operator=cos
  Cos{1..2,5,7} (4 alike) : Trigonometry
  Display : Display
  Gain : Gain  Gain=-1
  Gain1 : Gain  Gain=-1
  Ground{,1..3} (4 alike) : Ground
  Matrix Multiply : Product  Multiplication=Matrix(*)
  Reshape : Reshape  OutputDimensionality=Customize  OutputDimensions=[3,3]
  Reshape1 : Reshape  OutputDimensionality=Customize  OutputDimensions=[3,3]
  Vector Concatenate : Concatenate  NumInputs=9
  Vector Concatenate1 : Concatenate  NumInputs=9
  AL_N : Outport
  wires:
  Matrix Multiply/1 -> [AL_N], Display/1
  [AL_N] -> AL_N/1
  theta/1 -> [theta]
  Reshape/1 -> Matrix Multiply/1
  Reshape1/1 -> Matrix Multiply/2
  Cos/1 -> Vector Concatenate/1
  Cos1/1 -> Gain/1
  Gain/1 -> Vector Concatenate/2
  Ground/1 -> Vector Concatenate/3
  Cos2/1 -> Vector Concatenate/4
  Cos3/1 -> Vector Concatenate/5
  Ground1/1 -> Vector Concatenate/8, Vector Concatenate/7, Vector Concatenate/6
  Constant/1 -> Vector Concatenate/9
  [theta] -> Cos/1
  [theta] -> Cos1/1
  [theta] -> Cos2/1
  [theta] -> Cos3/1
  Vector Concatenate/1 -> Reshape/1
  Constant1/1 -> Vector Concatenate1/1
  Ground2/1 -> Vector Concatenate1/4, Vector Concatenate1/3, Vector Concatenate1/2
  Constant2/1 -> Cos4/1
  Cos4/1 -> Vector Concatenate1/5
  Constant3/1 -> Cos5/1
  Cos5/1 -> Gain1/1
  Gain1/1 -> Vector Concatenate1/6
  Ground3/1 -> Vector Concatenate1/7
  Constant4/1 -> Cos6/1
  Cos6/1 -> Vector Concatenate1/9
  Constant5/1 -> Cos7/1
  Cos7/1 -> Vector Concatenate1/8
  Vector Concatenate1/1 -> Reshape1/1

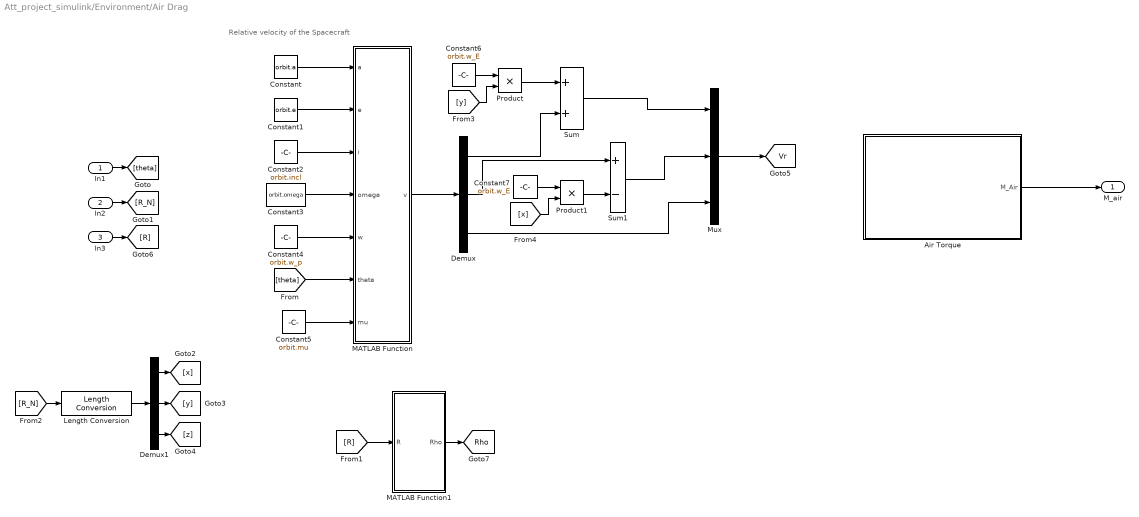
== system Att_project_simulink/Environment/Air Drag  ==
  note: Relative velocity of the Spacecraft
  In1 : Inport
  In2 : Inport  Port=2
  In3 : Inport  Port=3
  Air Torque : Subsystem
  Constant : Constant  Value=orbit.a
  Constant1 : Constant  Value=orbit.e
  Constant2 : Constant  Value=orbit.incl
  Constant3 : Constant  Value=orbit.omega
  Constant4 : Constant  Value=orbit.w_p
  Constant5 : Constant  Value=orbit.mu
  Constant6 : Constant  Value=orbit.w_E
  Constant7 : Constant  Value=orbit.w_E
  Demux : Demux  Outputs=3
  Demux1 : Demux  Outputs=3
  Length Conversion : aerolibconvert2/Length Conversion  IU=km  OU=m
  MATLAB Function : MATLAB Function  TreatAsAtomicUnit=on
  MATLAB Function1 : MATLAB Function  TreatAsAtomicUnit=on
  Mux : Mux  Inputs=3
  Product : Product
  Product1 : Product
  Sum : Sum
  Sum1 : Sum  Inputs=+-
  M_air : Outport
  tag scope: Rho=global, Vr=global
  wires:
  Constant5/1 -> MATLAB Function/7(mu)
  Constant4/1 -> MATLAB Function/5(w)
  Constant3/1 -> MATLAB Function/4(omega)
  Constant2/1 -> MATLAB Function/3(i)
  Constant1/1 -> MATLAB Function/2(e)
  Constant/1 -> MATLAB Function/1(a)
  In1/1 -> [theta]
  [theta] -> MATLAB Function/6(theta)
  In2/1 -> [R_N]
  MATLAB Function/1(v) -> Demux/1
  Demux/1 -> Sum/2
  Demux1/1 -> [x]
  Demux1/2 -> [y]
  Demux1/3 -> [z]
  Constant6/1 -> Product/1
  [y] -> Product/2
  Product/1 -> Sum/1
  Demux/2 -> Sum1/1
  Constant7/1 -> Product1/1
  [x] -> Product1/2
  Product1/1 -> Sum1/2
  Sum1/1 -> Mux/2
  Sum/1 -> Mux/1
  Demux/3 -> Mux/3
  In3/1 -> [R]
  [R] -> MATLAB Function1/1(R)
  MATLAB Function1/1(Rho) -> [Rho]
  Air Torque/1(M_Air) -> M_air/1
  Mux/1 -> [Vr]
  Length Conversion/1 -> Demux1/1
  [R_N] -> Length Conversion/1

== system Att_project_simulink/Environment/Magnetif Field Model ==
  R : Inport
  Rn : Inport  Port=2
  ThetaG0 : Inport  Port=3
  t : Inport  Port=4
  W_E : Inport  Port=5
  t0 : Inport  Port=6
  A_B/N : Inport  Port=7
  Constant : Constant  Value=13
  Constant1 : Constant  Value=g
  Constant2 : Constant  Value=h
  Constant3 : Constant  Value=K
  Constant7 : Constant  Value=m_para
  Cross Product : vrlib/Utilities/Cross Product
  Gain1 : Gain  Gain=1e-9
  Ground Track : Subsystem
  Integrator : Integrator  InitialConditionSource=external
  MATLAB Function : MATLAB Function  TreatAsAtomicUnit=on
  Matrix Multiply : Product  Multiplication=Matrix(*)
  Scope1 : Scope
  Scope3 : Scope
  Out1 : Outport
  b_N : Outport  Port=2
  b_B : Outport  Port=3
  wires:
  t0/1 -> Ground Track/5(t0)
  MATLAB Function/1(B) -> Gain1/1
  Ground Track/2(Lat) -> MATLAB Function/4(lat)
  Ground Track/1(Lon) -> MATLAB Function/1(long)
  t/1 -> Ground Track/3(t)
  Gain1/1 -> b_N/1, [b_N], Scope3/1
  ThetaG0/1 -> Integrator/2, Ground Track/2(ThetaG0)
  Rn/1 -> Ground Track/1(Rn)
  W_E/1 -> Integrator/1, Ground Track/4(W_E)
  A_B/N/1 -> Matrix Multiply/1
  [b_B] -> Cross Product/2
  Matrix Multiply/1 -> b_B/1, Scope1/1, [b_B]
  [b_N] -> Matrix Multiply/2
  Cross Product/1 -> Out1/1, [M_M]
  Constant7/1 -> Cross Product/1
  R/1 -> MATLAB Function/2(radius)
  Integrator/1 -> MATLAB Function/3(alpha_G)
  Constant1/1 -> MATLAB Function/5(g)
  Constant2/1 -> MATLAB Function/6(h)
  Constant3/1 -> MATLAB Function/7(K)
  Constant/1 -> MATLAB Function/9(N)
  Ground Track/3(R_norm) -> MATLAB Function/8(R)

== system Att_project_simulink/Environment/Rn ==
  theta : Inport
  R : Inport  Port=2
  Constant13 : Constant  Value=orbit.incl
  Constant14 : Constant  Value=orbit.incl
  Cos3 : Trigonometry  Operator=cos
  Cos4 : Trigonometry
  Cos5 : Trigonometry
  Mux2 : Mux  Inputs=3
  Product4 : Product
  Product5 : Product  Inputs=3
  Product6 : Product  Inputs=3
  Sin2 : Trigonometry  Operator=cos
  Sin3 : Trigonometry
  Rn : Outport
  wires:
  Constant14/1 -> Sin3/1
  Product6/1 -> [Rn_3]
  [theta] -> Cos4/1
  [Rn_1] -> Mux2/1
  Cos4/1 -> Product5/1
  [R] -> Product6/3
  [Rn_2] -> Mux2/2
  [R] -> Product4/2
  Mux2/1 -> Rn/1
  [theta] -> Cos5/1
  Sin3/1 -> Product6/2
  Cos5/1 -> Product6/1
  Product4/1 -> [Rn_1]
  Cos3/1 -> Product4/1
  [Rn_3] -> Mux2/3
  Sin2/1 -> Product5/2
  Constant13/1 -> Sin2/1
  Product5/1 -> [Rn_2]
  [R] -> Product5/3
  [theta] -> Cos3/1
  theta/1 -> [theta]
  R/1 -> [R]

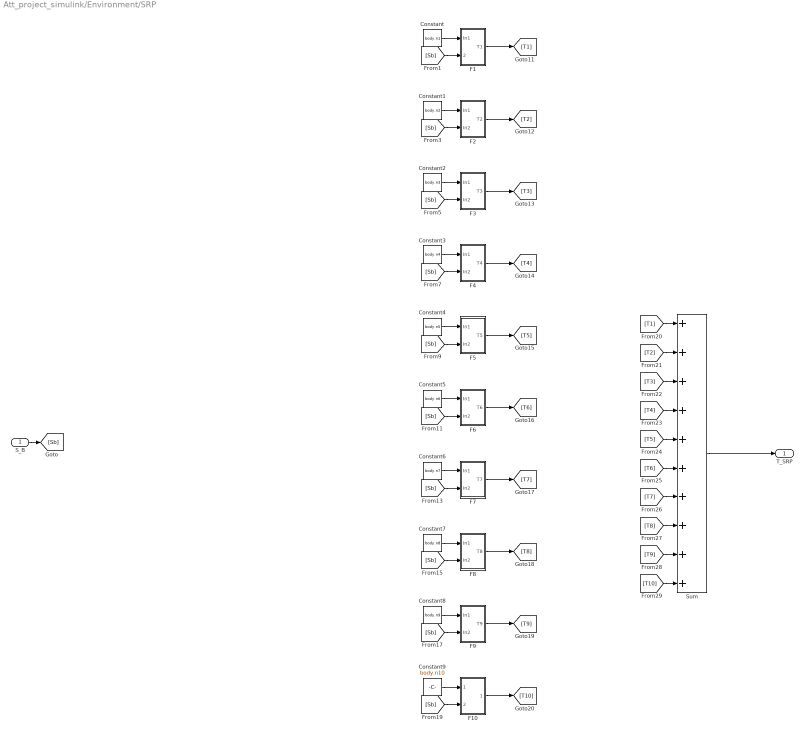
== system Att_project_simulink/Environment/SRP ==
  S_B : Inport
  Constant : Constant  Value=body.n1
  Constant1 : Constant  Value=body.n2
  Constant2 : Constant  Value=body.n3
  Constant3 : Constant  Value=body.n4
  Constant4 : Constant  Value=body.n5
  Constant5 : Constant  Value=body.n6
  Constant6 : Constant  Value=body.n7
  Constant7 : Constant  Value=body.n8
  Constant8 : Constant  Value=body.n9
  Constant9 : Constant  Value=body.n10
  F1 : Subsystem
  F10 : Subsystem
  F2 : Subsystem
  F3 : Subsystem
  F4 : Subsystem
  F5 : Subsystem
  F6 : Subsystem
  F7 : Subsystem
  F8 : Subsystem
  F9 : Subsystem
  Sum : Sum  Inputs=++++++++++
  T_SRP : Outport
  wires:
  S_B/1 -> [Sb]
  F1/1(T1) -> [T1]
  Constant/1 -> F1/1(In1)
  [Sb] -> F1/2(Input)
  F2/1(T2) -> [T2]
  Constant1/1 -> F2/1(In1)
  [Sb] -> F2/2(In2)
  [Sb] -> F3/2(In2)
  F3/1(T3) -> [T3]
  Constant2/1 -> F3/1(In1)
  [Sb] -> F4/2(In2)
  F4/1(T4) -> [T4]
  Constant3/1 -> F4/1(In1)
  [Sb] -> F5/2(In2)
  F5/1(T5) -> [T5]
  Constant4/1 -> F5/1(In1)
  [Sb] -> F6/2(In2)
  F6/1(T6) -> [T6]
  Constant5/1 -> F6/1(In1)
  [Sb] -> F7/2(In2)
  F7/1(T7) -> [T7]
  Constant6/1 -> F7/1(In1)
  [Sb] -> F8/2(In2)
  F8/1(T8) -> [T8]
  Constant7/1 -> F8/1(In1)
  [Sb] -> F9/2(In2)
  F9/1(T9) -> [T9]
  Constant8/1 -> F9/1(In1)
  [Sb] -> F10/2(In2)
  F10/1(T10) -> [T10]
  Constant9/1 -> F10/1(In1)
  [T10] -> Sum/10
  [T9] -> Sum/9
  [T8] -> Sum/8
  [T7] -> Sum/7
  [T6] -> Sum/6
  [T5] -> Sum/5
  [T4] -> Sum/4
  [T3] -> Sum/3
  [T2] -> Sum/2
  [T1] -> Sum/1
  Sum/1 -> T_SRP/1

== system Att_project_simulink/Environment/Sn ==
  t : Inport
  Constant15 : Constant  Value=orbit.n_sun
  Constant16 : Constant  Value=orbit.n_sun
  Constant17 : Constant  Value=orbit.eclip
  Constant18 : Constant  Value=orbit.n_sun
  Constant19 : Constant  Value=orbit.eclip
  Cos10 : Trigonometry  Operator=cos
  Cos6 : Trigonometry  Operator=cos
  Cos7 : Trigonometry
  Cos8 : Trigonometry
  Cos9 : Trigonometry
  Gain : Gain  Gain=Rs
  Gain1 : Gain  Gain=Rs
  Gain2 : Gain  Gain=Rs
  Mux3 : Mux  Inputs=3
  Product{7..11} (5 alike) : Product
  Scope : Scope
  Sn : Outport
  wires:
  Cos10/1 -> Product9/2
  [t] -> Product10/1
  [t] -> Product8/1
  Constant19/1 -> Cos7/1
  Constant18/1 -> Product10/2
  Product8/1 -> Cos8/1
  Product11/1 -> Gain2/1
  Cos8/1 -> Product9/1
  Constant15/1 -> Product7/2
  Product10/1 -> Cos9/1
  Mux3/1 -> Scope/1, Sn/1
  [t] -> Product7/1
  Cos9/1 -> Product11/1
  Cos7/1 -> Product11/2
  Product7/1 -> Cos6/1
  Cos6/1 -> Gain1/1
  Constant16/1 -> Product8/2
  Constant17/1 -> Cos10/1
  t/1 -> [t]
  Product9/1 -> Gain/1
  Gain/1 -> Mux3/2
  Gain1/1 -> Mux3/1
  Gain2/1 -> Mux3/3

== system Att_project_simulink/Environment/Subsystem ==
  Constant3 : Constant
  Constant4 : Constant  Value=orbit.e
  Constant5 : Constant  Value=orbit.n
  Constant6 : Constant
  Constant8 : Constant  Value=orbit.e
  Constant9 : Constant  Value=3/2
  Cos1 : Trigonometry  Operator=cos
  Divide : Product  Inputs=*/
  Integrator : Integrator  InitialCondition=1
  Power2 : Math  Operator=pow
  Product : Product
  Product1 : Product
  Square : Math  Operator=square
  Square1 : Math  Operator=square
  Sum2 : Sum
  Sum3 : Sum  Inputs=+-
  Theta : Outport
  wires:
  Product1/1 -> Divide/1
  Constant4/1 -> Product/1
  Constant8/1 -> Square/1
  Divide/1 -> Integrator/1
  Constant5/1 -> Product1/2
  Cos1/1 -> Product/2
  Power2/1 -> Divide/2
  Product/1 -> Sum2/2
  Square1/1 -> Product1/1
  Constant9/1 -> Power2/2
  Sum2/1 -> Square1/1
  Constant3/1 -> Sum2/1
  Square/1 -> Sum3/2
  Constant6/1 -> Sum3/1
  Sum3/1 -> Power2/1
  Integrator/1 -> Theta/1, Cos1/1

== system Att_project_simulink/Environment/Subsystem1 ==
  Theta : Inport
  Constant10 : Constant  Value=orbit.a
  Constant11 : Constant
  Constant12 : Constant  Value=orbit.e
  Constant5 : Constant
  Constant7 : Constant  Value=orbit.e
  Cos2 : Trigonometry  Operator=cos
  Divide1 : Product  Inputs=*/
  Product2 : Product
  Product3 : Product
  Scope : Scope
  Square2 : Math  Operator=square
  Sum4 : Sum  Inputs=+-
  Sum5 : Sum
  R : Outport
  wires:
  Sum4/1 -> Product2/1
  Cos2/1 -> Product3/2
  Product3/1 -> Sum5/2
  Theta/1 -> Cos2/1
  Square2/1 -> Sum4/2
  Constant7/1 -> Product3/1
  Constant11/1 -> Sum4/1
  Product2/1 -> Divide1/1
  Constant12/1 -> Square2/1
  Constant5/1 -> Sum5/1
  Constant10/1 -> Product2/2
  Sum5/1 -> Divide1/2
  Divide1/1 -> Scope/1, R/1

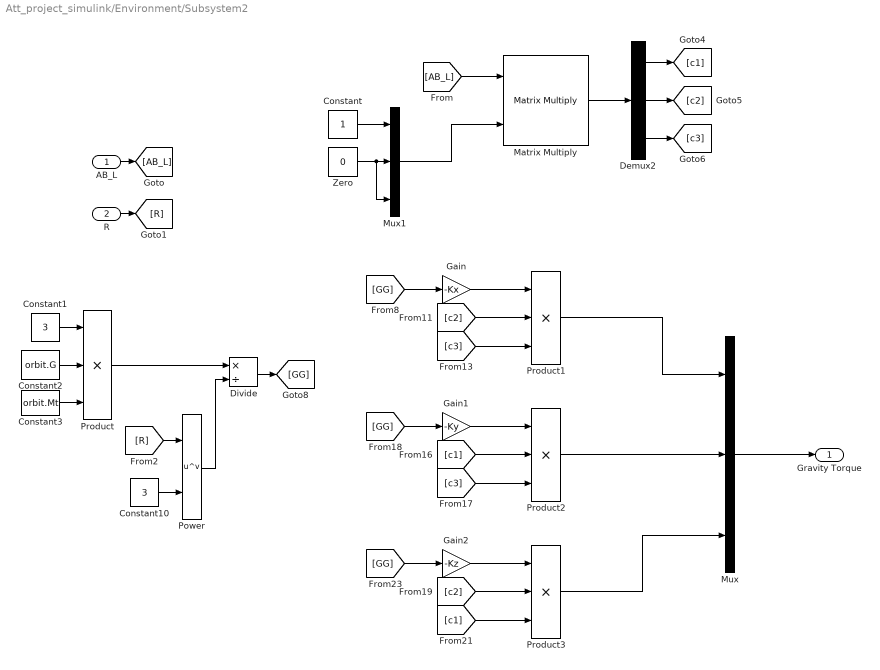
== system Att_project_simulink/Environment/Subsystem2 ==
  AB_L : Inport
  R : Inport  Port=2
  Constant : Constant
  Constant1 : Constant  Value=3
  Constant10 : Constant  Value=3
  Constant2 : Constant  Value=orbit.G
  Constant3 : Constant  Value=orbit.Mt
  Demux2 : Demux  Outputs=3
  Divide : Product  Inputs=*/
  Gain : Gain  Gain=-Kx
  Gain1 : Gain  Gain=-Ky
  Gain2 : Gain  Gain=-Kz
  Matrix Multiply : Product  Multiplication=Matrix(*)
  Mux : Mux  Inputs=3
  Mux1 : Mux  Inputs=3
  Power : Math  Operator=pow
  Product{,1..3} (4 alike) : Product  Inputs=3
  Zero : Constant  Value=0  OutDataTypeStr=Inherit: Inherit via back propagation
  Gravity Torque : Outport
  wires:
  [c3] -> Product2/3
  [GG] -> Gain/1
  [c2] -> Product1/2
  [AB_L] -> Matrix Multiply/1
  [c2] -> Product3/2
  [c3] -> Product1/3
  [GG] -> Gain2/1
  [c1] -> Product2/2
  Gain2/1 -> Product3/1
  Mux1/1 -> Matrix Multiply/2
  Gain/1 -> Product1/1
  Demux2/1 -> [c1]
  Zero/1 -> Mux1/3, Mux1/2
  Mux/1 -> Gravity Torque/1
  Gain1/1 -> Product2/1
  Matrix Multiply/1 -> Demux2/1
  Product2/1 -> Mux/2
  Product1/1 -> Mux/1
  Demux2/3 -> [c3]
  [GG] -> Gain1/1
  Product3/1 -> Mux/3
  [c1] -> Product3/3
  Constant/1 -> Mux1/1
  Demux2/2 -> [c2]
  AB_L/1 -> [AB_L]
  Constant10/1 -> Power/2
  Divide/1 -> [GG]
  [R] -> Power/1
  Product/1 -> Divide/1
  Power/1 -> Divide/2
  Constant3/1 -> Product/3
  Constant1/1 -> Product/1
  Constant2/1 -> Product/2
  R/1 -> [R]

== system Att_project_simulink/Environment/WB_L error ==
  AB_L : Inport
  wB : Inport  Port=2
  wL_N : Inport  Port=3
  Matrix Multiply1 : Product  Multiplication=Matrix(*)
  Sum : Sum  Inputs=+-
  attitude error : Outport
  wires:
  Matrix Multiply1/1 -> Sum/2
  [wL_N] -> Matrix Multiply1/2
  [AB_L] -> Matrix Multiply1/1
  Sum/1 -> attitude error/1
  AB_L/1 -> [AB_L]
  wL_N/1 -> [wL_N]
  wB/1 -> [wB]
  [wB] -> Sum/1

== system Att_project_simulink/Kynematics/DCM ==
  wB : Inport
  A_DCM : Scope
  Demux3 : Demux  Outputs=3
  Determinant of 3x3 Matrix : sharedutil/Determinant of 3x3 Matrix  aMode=aMode
  Determinant of 3x3 Matrix1 : sharedutil/Determinant of 3x3 Matrix  aMode=aMode
  Display : Display
  Gain{24..27} (4 alike) : Gain  Gain=-1
  Ground : Ground
  Ground1 : Ground
  Ground2 : Ground
  Integrator1 : Integrator  InitialCondition=A_R
  Matrix Multiply : Product  Multiplication=Matrix(*)
  Ortonormalization : Subsystem
  Reshape : Reshape  OutputDimensionality=Customize  OutputDimensions=[3,3]
  Scope : Scope
  Scope3 : Scope
  Scope7 : Scope
  To Workspace : ToWorkspace  VariableName=Adcm  SaveFormat=Timeseries  SampleTime=-1
  Vector Concatenate : Concatenate  NumInputs=9
  dcm : Outport
  wires:
  Demux3/2 -> Gain24/1, Vector Concatenate/7  "w_y"
  Determinant of 3x3 Matrix/1 -> Scope3/1
  Matrix Multiply/1 -> Integrator1/1
  Ground1/1 -> Vector Concatenate/5
  Ground2/1 -> Vector Concatenate/9
  Gain26/1 -> Vector Concatenate/8
  Ground/1 -> Vector Concatenate/1
  Vector Concatenate/1 -> Reshape/1
  Demux3/3 -> Vector Concatenate/2, Gain25/1  "w_z"
  wB/1 -> Demux3/1
  Gain24/1 -> Vector Concatenate/3
  Gain27/1 -> Matrix Multiply/1
  Gain25/1 -> Vector Concatenate/4
  Determinant of 3x3 Matrix1/1 -> Scope/1
  Demux3/1 -> Vector Concatenate/6, Gain26/1  "w_x"
  Reshape/1 -> Gain27/1
  Ortonormalization/1(dcm) -> Display/1, Determinant of 3x3 Matrix/1, To Workspace/1, Scope7/1, dcm/1
  Integrator1/1 -> Matrix Multiply/2, Ortonormalization/1(In1), A_DCM/1, Determinant of 3x3 Matrix1/1

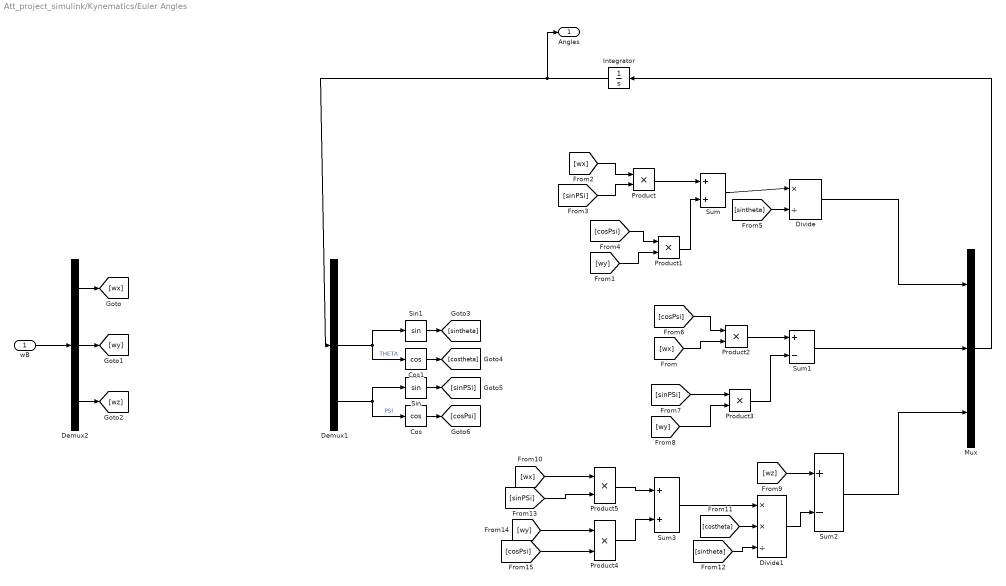
== system Att_project_simulink/Kynematics/Euler Angles ==
  wB : Inport
  Cos : Trigonometry  Operator=cos
  Cos1 : Trigonometry  Operator=cos
  Demux1 : Demux  Outputs=3
  Demux2 : Demux  Outputs=3
  Divide : Product  Inputs=*/
  Divide1 : Product  Inputs=**/
  Integrator : Integrator  InitialCondition=[phi0, theta0,psi0]
  Mux : Mux  Inputs=3
  Product{,1..5} (6 alike) : Product
  Sin : Trigonometry
  Sin1 : Trigonometry
  Sum : Sum
  Sum1 : Sum  Inputs=+-
  Sum2 : Sum  Inputs=+-
  Sum3 : Sum
  Angles : Outport
  wires:
  Demux2/3 -> [wz]
  Demux2/2 -> [wy]
  Demux2/1 -> [wx]
  wB/1 -> Demux2/1
  Demux1/2 -> Cos1/1, Sin1/1  "THETA"
  Demux1/3 -> Cos/1, Sin/1  "PSI"
  Cos1/1 -> [costheta]
  Cos/1 -> [cosPsi]
  Sin/1 -> [sinPSi]
  Sin1/1 -> [sintheta]
  Sum/1 -> Divide/1
  Product/1 -> Sum/1
  [wx] -> Product/1
  [sinPSi] -> Product/2
  [cosPsi] -> Product1/1
  [wy] -> Product1/2
  Product1/1 -> Sum/2
  [sintheta] -> Divide/2
  [cosPsi] -> Product2/1
  [wx] -> Product2/2
  Product2/1 -> Sum1/1
  [sinPSi] -> Product3/1
  [wy] -> Product3/2
  Product3/1 -> Sum1/2
  [wz] -> Sum2/1
  Product4/1 -> Sum3/2
  Product5/1 -> Sum3/1
  [wx] -> Product5/1
  Sum3/1 -> Divide1/1
  Divide1/1 -> Sum2/2
  [costheta] -> Divide1/2
  [sintheta] -> Divide1/3
  [sinPSi] -> Product5/2
  [wy] -> Product4/1
  [cosPsi] -> Product4/2
  Sum1/1 -> Mux/2
  Divide/1 -> Mux/1
  Sum2/1 -> Mux/3
  Mux/1 -> Integrator/1
  Integrator/1 -> Angles/1, Demux1/1

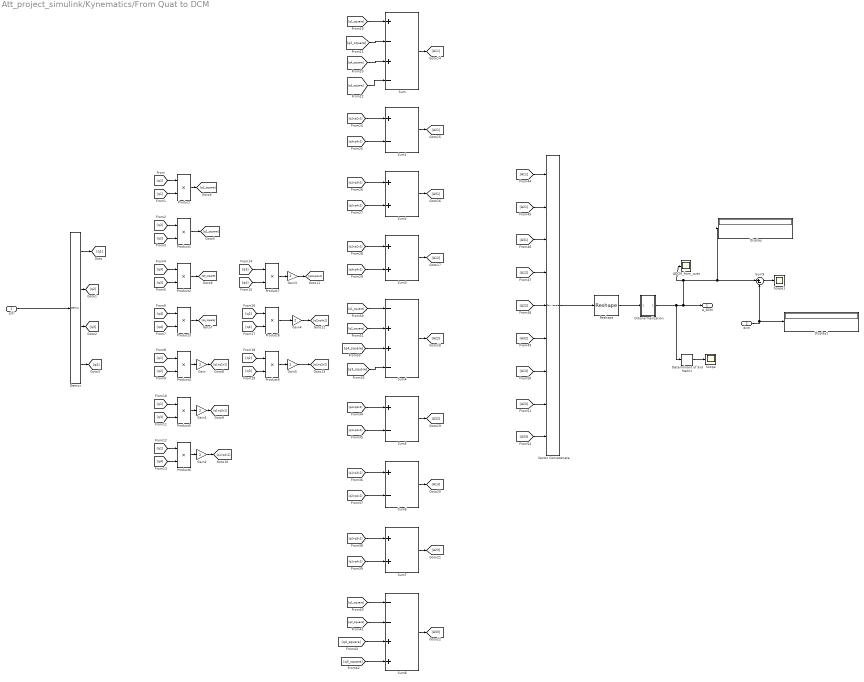
== system Att_project_simulink/Kynematics/From Quat to DCM ==
  q(t) : Inport
  dcm : Inport  Port=2
  ADCM_from_quat : Scope
  Demux : Demux
  Determinant of 3x3 Matrix : sharedutil/Determinant of 3x3 Matrix  aMode=aMode
  Display : Display
  Display1 : Display
  Gain{,1..5} (6 alike) : Gain  Gain=2
  Ortonormalization : Subsystem
  Product{,1..9} (10 alike) : Product
  Reshape : Reshape  OutputDimensionality=Customize  OutputDimensions=[3,3]
  Scope : Scope
  Scope1 : Scope
  Sum : Sum  Inputs=+-+-
  Sum1 : Sum  Inputs=+-
  Sum2 : Sum
  Sum3 : Sum
  Sum4 : Sum  Inputs=-++-
  Sum5 : Sum  Inputs=+-
  Sum6 : Sum  Inputs=+-
  Sum7 : Sum
  Sum8 : Sum  Inputs=--++
  Sum9 : Sum  Inputs=|+-
  Vector Concatenate : Concatenate  NumInputs=9
  A_DCM : Outport
  wires:
  [q1] -> Product/1
  Demux/2 -> [q2]
  [q1] -> Product/2
  [q2] -> Product1/1
  [q2] -> Product1/2
  [q3] -> Product2/1
  [q3] -> Product2/2
  [q4] -> Product3/1
  [q4] -> Product3/2
  Demux/3 -> [q3]
  [q1] -> Product4/1
  [q2] -> Product4/2
  [q1] -> Product5/1
  [q3] -> Product5/2
  [q1] -> Product6/1
  [q4] -> Product6/2
  [q3] -> Product7/1
  [q4] -> Product7/2
  [q2] -> Product8/1
  [q4] -> Product8/2
  [q2] -> Product9/1
  [q3] -> Product9/2
  Product/1 -> [q1_square]
  [q1_square] -> Sum/1
  Product1/1 -> [q2_square]
  Product2/1 -> [q3_square]
  Product3/1 -> [q4_square]
  [q2_square] -> Sum/2
  [q3_square] -> Sum/4
  [q4_square] -> Sum/3
  Gain/1 -> [q1xq2x2]
  Product4/1 -> Gain/1
  Gain1/1 -> [q1xq3x2]
  Product5/1 -> Gain1/1
  Gain2/1 -> [q1xq4x2]
  Product6/1 -> Gain2/1
  Product9/1 -> Gain5/1
  Gain5/1 -> [q2xq3x2]
  Gain4/1 -> [q2xq4x2]
  Product8/1 -> Gain4/1
  Gain3/1 -> [q3xq4x2]
  Product7/1 -> Gain3/1
  [q1xq2x2] -> Sum1/1
  [q3xq4x2] -> Sum1/2
  [q1xq3x2] -> Sum2/1
  [q2xq4x2] -> Sum2/2
  [q3xq4x2] -> Sum3/2
  [q1xq2x2] -> Sum3/1
  [q1_square] -> Sum4/1
  [q2_square] -> Sum4/2
  [q4_square] -> Sum4/3
  [q3_square] -> Sum4/4
  [q1xq4x2] -> Sum5/2
  [q2xq3x2] -> Sum5/1
  [q2xq4x2] -> Sum6/2
  [q1xq3x2] -> Sum6/1
  [q2xq3x2] -> Sum7/1
  [q1xq4x2] -> Sum7/2
  [q2_square] -> Sum8/2
  [q3_square] -> Sum8/4
  [q1_square] -> Sum8/1
  [q4_square] -> Sum8/3
  Sum/1 -> [A11]
  Sum1/1 -> [A21]
  Sum2/1 -> [A31]
  Sum3/1 -> [A12]
  Sum4/1 -> [A22]
  Sum5/1 -> [A32]
  Sum6/1 -> [A13]
  Sum7/1 -> [A23]
  Sum8/1 -> [A33]
  [A11] -> Vector Concatenate/1
  [A21] -> Vector Concatenate/2
  [A31] -> Vector Concatenate/3
  [A12] -> Vector Concatenate/4
  [A22] -> Vector Concatenate/5
  [A32] -> Vector Concatenate/6
  [A13] -> Vector Concatenate/7
  [A23] -> Vector Concatenate/8
  [A33] -> Vector Concatenate/9
  Vector Concatenate/1 -> Reshape/1
  Determinant of 3x3 Matrix/1 -> Scope/1
  Reshape/1 -> Ortonormalization/1(In1)
  Sum9/1 -> Scope1/1
  dcm/1 -> Sum9/2, Display1/1
  Ortonormalization/1(dcm) -> ADCM_from_quat/1, Display/1, Sum9/1, A_DCM/1, Determinant of 3x3 Matrix/1
  Demux/4 -> [q4]
  Demux/1 -> [q1]
  q(t)/1 -> Demux/1
